simulink model "compstate"  (R2017a)
settings: Solver=FixedStepDiscrete  StartTime=0.0  StopTime=30.0  FixedStep=0.1  RelTol=1e-3  EnableMultiTasking=on
settings Model: NumberOfSteps=10  Creator=thr  LastModifiedBy=thr
settings SolverCC: AutoInsertRateTranBlk=on
settings DataIOCC: LimitDataPoints=on
settings OptimizationCC: LifeSpan=inf
settings DebuggingCC: AllowSymbolicDim=off  SFUnexpectedBacktrackingDiag=warning  SFNoUnconditionalDefaultTransitionDiag=warning  SFExecutionAtInitializationDiag=none
settings GRTTargetCC: TargetLangStandard=C89/C90 (ANSI)  GeneratePreprocessorConditionals=Disable all
settings ConfigComp: CovMetricSettings=dw  CovHtmlReporting=on  CovSaveCumulativeToWorkspaceVar=on  CovSaveSingleToWorkspaceVar=on  CovShowResultsExplorer=off  CovExternalEMLEnable=off  CovSFcnEnable=off

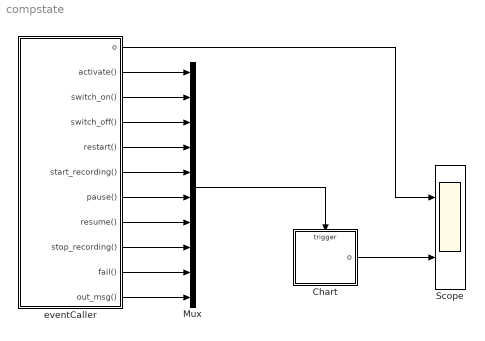
== system compstate ==
  Chart : Stateflow chart  TreatAsAtomicUnit=on
  Mux : Mux  Inputs=10
  Scope : Scope  NumInputPorts=2
  eventCaller : Stateflow chart  TreatAsAtomicUnit=on
  wires:
  Mux/1 -> Chart/Trigger
  Chart/1(o) -> Scope/2
  eventCaller/1(o) -> Scope/1
  eventCaller/11(out_msg()) -> Mux/10
  eventCaller/10(fail()) -> Mux/9
  eventCaller/9(stop_recording()) -> Mux/8
  eventCaller/8(resume()) -> Mux/7
  eventCaller/7(pause()) -> Mux/6
  eventCaller/6(start_recording()) -> Mux/5
  eventCaller/5(restart()) -> Mux/4
  eventCaller/4(switch_off()) -> Mux/3
  eventCaller/3(switch_on()) -> Mux/2
  eventCaller/2(activate()) -> Mux/1

== stateflow chart compstate/eventCaller ==
  state A
    entry: o = 1;
    activate
  state B
    entry: o = 2;
    switch_on
  state C
    entry: o = 3;
    start_recording
  state F
    entry: o = 6;
    stop_recording
  state E
    entry: o = 5;
    resume
  state D
    entry: o = 4;
    pause
  state G
    entry: o = 7;
    start_recording
  state H
    entry: o = 8;
    pause
  state I
    entry: o = 9;
    stop_recording
  state L
    entry: o = 12;
    restart
  state K
    entry: o = 11;
    fail
  state J
    entry: o = 10;
    start_recording
  state M
    entry: o = 13;
    switch_off
  (default) -> A
  A -> B : after(1, sec)
  B -> C : after(1, sec)
  C -> D : after(1, sec)
  E -> F : after(1, sec)
  D -> E : after(1, sec)
  F -> G : after(1, sec)
  G -> H : after(1, sec)
  H -> I : after(1, sec)
  I -> J : after(1, sec)
  K -> L : after(1, sec)
  J -> K : after(1, sec)
  L -> M : after(1, sec)
  data: o output int32
  events: activate output FUNCTION_CALL_EVENT; switch_on output FUNCTION_CALL_EVENT; switch_off output FUNCTION_CALL_EVENT; restart output FUNCTION_CALL_EVENT; start_recording output FUNCTION_CALL_EVENT; pause output FUNCTION_CALL_EVENT; resume output FUNCTION_CALL_EVENT; stop_recording output FUNCTION_CALL_EVENT; fail output FUNCTION_CALL_EVENT; out_msg output FUNCTION_CALL_EVENT

== stateflow chart compstate/Chart ==
  state ON
    entry: o = 1
    state READY
      entry: o = 5
    state RECORDING
      entry: o = 7
    state PAUSED
      entry: o = 9
    (default) -> READY
    READY -> RECORDING : start_recording
    RECORDING -> READY [order 3] : stop_recording
    PAUSED -> READY [order 2] : stop_recording
    PAUSED -> RECORDING [order 1] : resume
    RECORDING -> PAUSED [order 1] : pause
  state OFF
    entry: o = 0
  state FAULTY
    entry: o = 3
  (default) -> OFF : activate
  OFF -> ON : switch_on
  ON -> OFF : switch_off
  FAULTY -> READY : restart
  RECORDING -> FAULTY [order 2] : fail
  data: o output double
  events: activate input FUNCTION_CALL_EVENT; switch_on input FUNCTION_CALL_EVENT; switch_off input FUNCTION_CALL_EVENT; restart input FUNCTION_CALL_EVENT; start_recording input FUNCTION_CALL_EVENT; pause input FUNCTION_CALL_EVENT; resume input FUNCTION_CALL_EVENT; stop_recording input FUNCTION_CALL_EVENT; fail input FUNCTION_CALL_EVENT; out_msg input FUNCTION_CALL_EVENT
